simulink model "pend"  (Simulink 9.1)
settings: Solver=VariableStepAuto  StartTime=0.0  StopTime=tf  RelTol=1e-3
values from neighbouring files (symbols this model uses):
  C = [B_0, - l_1*m_1*theta1_p(k)*sin(theta1(k)) - l_1*m_2*theta1_p(k)*sin(theta1(k)) - l_1*m_3*theta1_p(k)*sin(theta1(k)), - l_2*m_2*theta2_p(k)*sin(theta2(k)) - l_2*m_3*theta2_p(k)*sin(theta2(k)), -l_3*m_3*theta3_p(k)*sin(theta3(k)) ... (first row only)    [DINAMICA_PENDULO_TRIPLE_INVERTIDO.m]    (also in PENDULO_DOBLE_INVERTIDO_MODELO.m = [B_0, - l_1*m_1*theta1_p(k)*sin(theta1(k)) - l_1*m_2*theta1_; VALIDACION_MODELO_MATEMATICO_PENDULO_DOBLE_INVERTIDO.m = [0, - l_1*m_1*theta1_p(k)*sin(theta1(k)) - l_1*m_2*theta1_p(; VALIDACION_MODELO_MATEMATICO_PENDULO_SIMPLE_INVERTIDO.m = [0, -l_1*m_1*theta1_p(k)*sin(theta1(k)); 0, 0]; pendulum.m = 5)
  g = 9.8    [CONTROL_PENDULO_INVERTIDO_VALIDACION.m]    (also in DINAMICA_PENDULO_TRIPLE_INVERTIDO.m; PENDULO_DOBLE_INVERTIDO_MODELO.m; PENDULO_INVERTIDO_CONTROL.m; VALIDACION_MODELO_MATEMATICO_PENDULO_DOBLE_INVERTIDO.m)
  L = 1.0    (= 1)    [pendulum.m]
  L2 = 1.0    (= 1)    [pendulum.m]
  m = 1.0    (= 1)    [pendulum.m]
  m2 = 1.0    (= 1)    [pendulum.m]
undefined symbols (not defined in the file or in its folder): magnitude
settings Model: Creator=DELL  LastModifiedBy=DELL
settings DataIOCC: SaveFormat=Dataset
settings OptimizationCC: LifeSpan=auto
settings DebuggingCC: UnderspecifiedInitializationDetection=Simplified  MergeDetectMultiDrivingBlocksExec=error  SFUnexpectedBacktrackingDiag=error  SFNoUnconditionalDefaultTransitionDiag=error  SFExecutionAtInitializationDiag=warning
settings HardwareCC: ProdBitPerPointer=64  ProdBitPerSizeT=64  ProdBitPerPtrDiffT=64  ProdLargestAtomicFloat=Float  ProdIntDivRoundTo=Zero  ProdEndianess=LittleEndian  ProdWordSize=64  ProdHWDeviceType=Intel->x86-64 (Windows64)
settings ModelReferenceCC: PropagateSignalLabelsOutOfModel=on
settings CodeAppCC: StateflowObjectComments=off
settings GRTTargetCC: TargetLangStandard=C99 (ISO)  CombineOutputUpdateFcns=on  GRTInterface=off
settings ConfigComp: CovMetricSettings=dwe  CovHtmlReporting=off  CovSaveCumulativeToWorkspaceVar=off  CovSaveSingleToWorkspaceVar=off  CovExternalEMLEnable=on

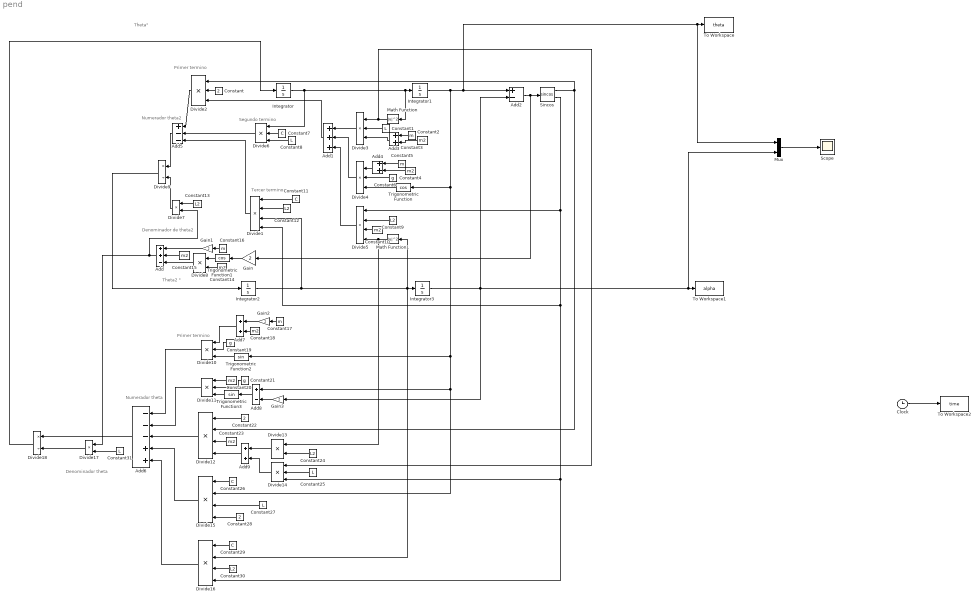
== system pend ==
  note: Denominador theta
  note: Primer termino
  note: Tercer termino
  note: Segundo termino
  note: Primer termino
  note: Numerador theta
  note: Denominador de theta2
  note: Numerador theta2
  note: Theta2 "
  note: Theta"
  Add : Sum  Inputs=++-
  Add1 : Sum  Inputs=+++
  Add2 : Sum  Inputs=+-
  Add{3..4,7,9} (4 alike) : Sum
  Add5 : Sum  Inputs=+--
  Add6 : Sum  Inputs=---++
  Add8 : Sum  Inputs=+-
  Clock : Clock
  Constant : Constant  Value=2
  Constant{1,8,25,27,31} (5 alike) : Constant  Value=L
  Constant{2,4,10,14..15,18,20,23} (8 alike) : Constant  Value=m2
  Constant{7,11,26,29} (4 alike) : Constant  Value=C
  Constant{9,12..13,24,30} (5 alike) : Constant  Value=L2
  Constant{3,5,16..17} (4 alike) : Constant  Value=m
  Constant19 : Constant  Value=g
  Constant21 : Constant  Value=g
  Constant22 : Constant  Value=2
  Constant28 : Constant  Value=2
  Constant6 : Constant  Value=g
  Divide{1,5,12,15..16} (5 alike) : Product  Inputs=****
  Divide{2..4,6,10..11,14} (7 alike) : Product  Inputs=***
  Divide{7..8,13,17} (4 alike) : Product  Inputs=**
  Divide18 : Product  Inputs=*/
  Divide9 : Product  Inputs=*/
  Gain{,1..3} (4 alike) : Gain  Gain=2
  Integrator : Integrator  InitialCondition=3
  Integrator1 : Integrator
  Integrator2 : Integrator  InitialCondition=3
  Integrator3 : Integrator
  Math Function : Math  Operator=magnitude^2  SaturateOnIntegerOverflow=on
  Math Function1 : Math  Operator=magnitude^2  SaturateOnIntegerOverflow=on
  Mux : Mux  Inputs=2
  Scope : Scope
  Sincos : Trigonometry  Operator=sincos
  To Workspace : ToWorkspace  VariableName=theta  SampleTime=-1
  To Workspace1 : ToWorkspace  VariableName=alpha  SampleTime=-1
  To Workspace2 : ToWorkspace  VariableName=time  SampleTime=-1
  Trigonometric Function : Trigonometry  Operator=cos
  Trigonometric Function1 : Trigonometry  Operator=cos
  Trigonometric Function2 : Trigonometry
  Trigonometric Function3 : Trigonometry
  wires:
  Integrator2/1 -> Integrator3/1, Math Function1/1, Divide16/2, Divide1/3
  Integrator/1 -> Divide6/1, Math Function/1, Integrator1/1
  Integrator3/1 -> Mux/2, To Workspace1/1, Gain3/1, Add2/2
  Integrator1/1 -> Trigonometric Function/1, Trigonometric Function2/1, Divide15/2, Add8/1, Mux/1, To Workspace/1, Add2/1
  Math Function/1 -> Divide14/1, Divide3/1
  Constant1/1 -> Divide3/2
  Add3/1 -> Divide3/3
  Constant3/1 -> Add3/1
  Constant2/1 -> Add3/2
  Divide3/1 -> Add1/1
  Constant4/1 -> Add4/2
  Constant5/1 -> Add4/1
  Add4/1 -> Divide4/1
  Constant6/1 -> Divide4/2
  Constant/1 -> Divide2/2
  Divide4/1 -> Add1/2
  Constant9/1 -> Divide5/2
  Math Function1/1 -> Divide13/1, Divide5/4
  Constant10/1 -> Divide5/3
  Trigonometric Function/1 -> Divide4/3
  Add2/1 -> Gain/1, Sincos/1
  Sincos/1 -> Divide12/2, Divide2/1
  Sincos/2 -> Divide16/4, Divide14/3, Divide1/4, Divide5/1
  Divide5/1 -> Add1/3
  Add1/1 -> Divide2/3
  Constant8/1 -> Divide6/3
  Constant7/1 -> Divide6/2
  Constant12/1 -> Divide1/2
  Constant11/1 -> Divide1/1
  Divide6/1 -> Add5/2
  Divide1/1 -> Add5/3
  Divide2/1 -> Add5/1
  Constant13/1 -> Divide7/1
  Gain/1 -> Trigonometric Function1/1
  Trigonometric Function1/1 -> Divide8/1
  Constant14/1 -> Divide8/2
  Divide8/1 -> Add/3
  Constant15/1 -> Add/2
  Constant16/1 -> Gain1/1
  Gain1/1 -> Add/1
  Add/1 -> Divide17/1, Divide7/2
  Add5/1 -> Divide9/1
  Divide7/1 -> Divide9/2
  Divide9/1 -> Integrator2/1
  Divide10/1 -> Add6/1
  Constant17/1 -> Gain2/1
  Gain2/1 -> Add7/1
  Add7/1 -> Divide10/1
  Constant18/1 -> Add7/2
  Constant19/1 -> Divide10/2
  Trigonometric Function2/1 -> Divide10/3
  Divide11/1 -> Add6/2
  Constant20/1 -> Divide11/1
  Constant21/1 -> Divide11/2
  Trigonometric Function3/1 -> Divide11/3
  Add8/1 -> Trigonometric Function3/1
  Gain3/1 -> Add8/2
  Divide12/1 -> Add6/3
  Constant22/1 -> Divide12/1
  Constant23/1 -> Divide12/3
  Add9/1 -> Divide12/4
  Divide13/1 -> Add9/1
  Constant24/1 -> Divide13/2
  Divide14/1 -> Add9/2
  Constant25/1 -> Divide14/2
  Divide15/1 -> Add6/4
  Constant26/1 -> Divide15/1
  Constant27/1 -> Divide15/3
  Constant28/1 -> Divide15/4
  Divide16/1 -> Add6/5
  Constant29/1 -> Divide16/1
  Constant30/1 -> Divide16/3
  Constant31/1 -> Divide17/2
  Add6/1 -> Divide18/1
  Divide17/1 -> Divide18/2
  Divide18/1 -> Integrator/1
  Mux/1 -> Scope/1
  Clock/1 -> To Workspace2/1
